simulink model "ros_test"  (R2019a)
settings: Solver=VariableStepAuto  StartTime=0.0  StopTime=inf  RelTol=1e-3
libraries: robotlib x2, aerolibanimutils x1
settings Model: Creator=flying  LastModifiedBy=flying

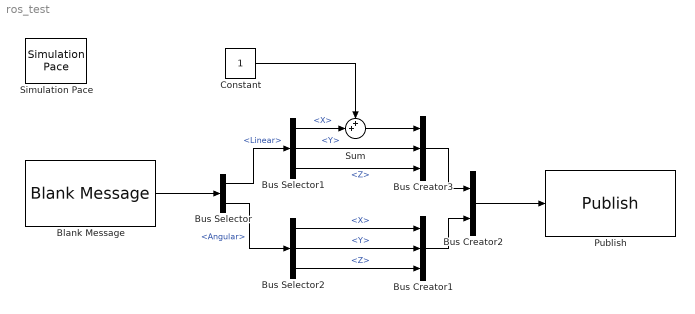
== system ros_test ==
  Blank Message : robotlib/Blank Message  messageClass=Message  entityType=geometry_msgs/Twist  messageType=geometry_msgs/Twist  SampleTime=1
      settings: SourceProductBaseCode=RO
  Bus Creator1 : BusCreator  Inputs=3  OutDataTypeStr=Bus: SL_Bus_ros_test_geometry_msgs_Vector3  NonVirtualBus=on
      settings: InheritFromInputs=off
  Bus Creator2 : BusCreator  Inputs=2  OutDataTypeStr=Bus: SL_Bus_ros_test_geometry_msgs_Twist  NonVirtualBus=on
      settings: InheritFromInputs=off
  Bus Creator3 : BusCreator  Inputs=3  OutDataTypeStr=Bus: SL_Bus_ros_test_geometry_msgs_Vector3  NonVirtualBus=on
      settings: InheritFromInputs=off
  Bus Selector : BusSelector  OutputSignals=Linear,Angular
  Bus Selector1 : BusSelector  OutputSignals=X,Y,Z
  Bus Selector2 : BusSelector  OutputSignals=X,Y,Z
  Constant : Constant
  Publish : robotlib/Publish  topicSource=Specify your own  topic=/test_twist  messageType=geometry_msgs/Twist  messageQueueLength=1
      settings: SourceProductBaseCode=RO
  Simulation Pace : aerolibanimutils/Simulation Pace  SimulationPace=1  SleepMode=Auto  OutputPaceError=off  SampleTime=1/30
  Sum : Sum  Inputs=++|
  wires:
  Bus Selector/2 -> Bus Selector2/1  "<Angular>"
  Blank Message/1 -> Bus Selector/1
  Bus Selector/1 -> Bus Selector1/1  "<Linear>"
  Bus Selector1/2 -> Bus Creator3/2  "<Y>"
  Bus Selector1/3 -> Bus Creator3/3  "<Z>"
  Bus Selector2/1 -> Bus Creator1/1  "<X>"
  Bus Selector2/2 -> Bus Creator1/2  "<Y>"
  Bus Selector2/3 -> Bus Creator1/3  "<Z>"
  Bus Creator3/1 -> Bus Creator2/1
  Bus Creator1/1 -> Bus Creator2/2
  Bus Creator2/1 -> Publish/1
  Sum/1 -> Bus Creator3/1
  Bus Selector1/1 -> Sum/2  "<X>"
  Constant/1 -> Sum/1
